simulink model "batteryCellModelling"  (R2024a)
settings: Solver=VariableStepAuto  StartTime=0.0  StopTime=3600  RelTol=1e-3
libraries: fl_lib x7, nesl_utility x4, batteryecm_lib x1
settings Model: Creator=KimoStore  LastModifiedBy=KimoStore
settings ModelReferenceCC: EnableRefExpFcnMdlSchedulingChecks=on
settings RTWCC: GPUComputeCapability=3.5

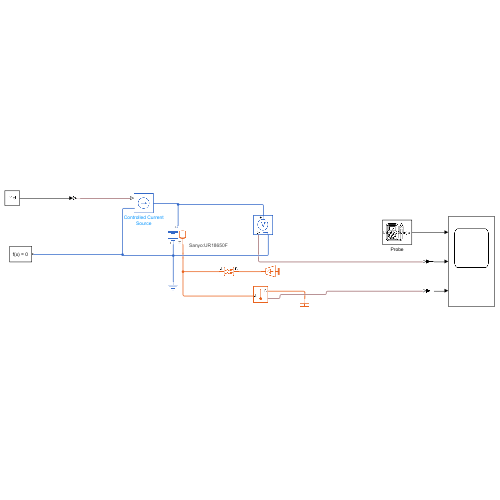
[thumbnail: Simulink's stored preview of the top-level diagram]
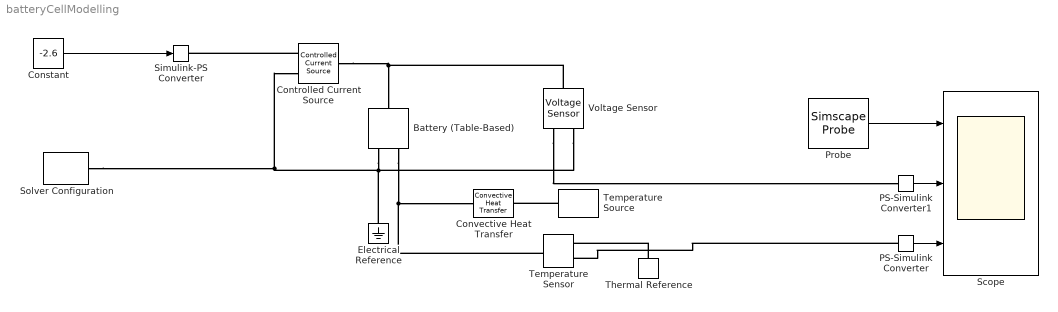
== system batteryCellModelling ==
  Battery (Table-Based) : batteryecm_lib/Battery (Table-Based)  Tag={'toolbox/physmod/battery/shared_library/m/batteryecm_lib_parts';'Battery__Table_Based_/Sanyo/UR18650F.xml'}  SOC_vec=[0 0.01 0.02 0.03 0.04 0.05 0.06 0.07 0.08 0.09 0.1 0.11 0.12 0.13 0.14 0.15 0.16 0.17 0.18 0.19 0.2 0.21 0.22 0.23 0.24 0.25 0.26 0.27 0.28 0.29 0.3 0.31 0.32 0.33 0.34 0.35 0.36 0.37 0.38 0.39 0.4 0.41 0.42 0.43 0.44 0.45 0.46 0.47 0.48 0.49 0.5 0.51 0.52 0.53 0.54 0.55 0.56 0.57 0.58 0.59 0.6 0.61 0.62 0.63 0.64 0.65 0.66 0.67 0.68 0.69 0.7 0.71 0.72 0.73 0.74 0.75 0.76 0.77 0.78 0.79 0.8 0.81 0.82 0.83 0.84 0.85 0.86 0.87 0.88 0.89 0.9 0.91 0.92 0.93 0.94 0.95 0.96 0.97 0.98 0.99 1]  T_dependence=simscape.enum.tablebattery.temperature_dependence.yes  prm_dir=simscape.enum.tablebattery.prm_dir.noCurrentDirectionality  T_vec=[-20 -10 0 20 40] degC  V0_mat=[3.0106 3.0106 3.0106 3.0106 3.0106;3.47625 3.47625 3.47625 3.47625 3.47625;3.60079 3.60079 3.60079 3.60079 3.60079;3.6231 3.6231 3.6231 3.6231 3.6231;3.64643 3.64643 3.64643 3.64643 3.64643;3.64894 3.64894 3.64894 3.64894 3.64894;3.65685 3.65685 3.65685 3.65685 3.65685;3.66356 3.66356 3.66356 3.66356 3.66356;3.66315 3.66315 3.66315 3.66315 3.66315;3.6671 3.6671 3.6671 3.6671 3.6671;3.67003 3.67003 3.67003 3.67003 3.67003;3.67239 3.67239 3.67239 3.67239 3.67239;3.67782 3.67782 3.67782 3.67782 3.67782;3.68366 3.68366 3.68366 3.68366 3.68366;3.68873 3.68873 3.68873 3.68873 3.68873;3.6931 3.6931 3.6931 3.6931 3.6931;3.69764 3.69764 3.69764 3.69764 3.69764;3.70218 3.70218 3.70218 3.70218 3.70218;3.70672 3.70672 3.70672 3.70672 3.70672;3.7109 3.7109 3.7109 3.7109 3.7109;3.71581 3.71581 3.71581 3.71581 3.71581;3.71846 3.71846 3.71846 3.71846 3.71846;3.7202 3.7202 3.7202 3.7202 3.7202;3.72195 3.72195 3.72195 3.72195 3.72195;3.7237 3.7237 3.7237 3.7237 3.7237;3.72544 3.72544 3.72544 3.72544 3.72544;3.72714 3.72714 3.72714 3.72714 3.72714;3.72856 3.72856 3.72856 3.72856 3.72856;3.72994 3.72994 3.72994 3.72994 3.72994;3.73135 3.73135 3.73135 3.73135 3.73135;3.7329 3.7329 3.7329 3.7329 3.7329;3.73481 3.73481 3.73481 3.73481 3.73481;3.73671 3.73671 3.73671 3.73671 3.73671;3.73861 3.73861 3.73861 3.73861 3.73861;3.74052 3.74052 3.74052 3.74052 3.74052;3.74259 3.74259 3.74259 3.74259 3.74259;3.74529 3.74529 3.74529 3.74529 3.74529;3.74799 3.74799 3.74799 3.74799 3.74799;3.75066 3.75066 3.75066 3.75066 3.75066;3.75332 3.75332 3.75332 3.75332 3.75332;3.75598 3.75598 3.75598 3.75598 3.75598;3.75851 3.75851 3.75851 3.75851 3.75851;3.76097 3.76097 3.76097 3.76097 3.76097;3.76344 3.76344 3.76344 3.76344 3.76344;3.76591 3.76591 3.76591 3.76591 3.76591;3.76898 3.76898 3.76898 3.76898 3.76898;3.77223 3.77223 3.77223 3.77223 3.77223;3.77526 3.77526 3.77526 3.77526 3.77526;3.7786 3.7786 3.7786 3.7786 3.7786;3.78229 3.78229 3.78229 3.78229 3.78229;3.78598 3.78598 3.78598 3.78598 3.78598;3.78967 3.78967 3.78967 3.78967 3.78967;3.79335 3.79335 3.79335 3.79335 3.79335;3.79704 3.79704 3.79704 3.79704 3.79704;3.80111 3.80111 3.80111 3.80111 3.80111;3.80653 3.80653 3.80653 3.80653 3.80653;3.81239 3.81239 3.81239 3.81239 3.81239;3.81825 3.81825 3.81825 3.81825 3.81825;3.8241 3.8241 3.8241 3.8241 3.8241;3.82996 3.82996 3.82996 3.82996 3.82996;3.83582 3.83582 3.83582 3.83582 3.83582;3.84168 3.84168 3.84168 3.84168 3.84168;3.84738 3.84738 3.84738 3.84738 3.84738;3.85296 3.85296 3.85296 3.85296 3.85296;3.85814 3.85814 3.85814 3.85814 3.85814;3.86321 3.86321 3.86321 3.86321 3.86321;3.86829 3.86829 3.86829 3.86829 3.86829;3.87336 3.87336 3.87336 3.87336 3.87336;3.87896 3.87896 3.87896 3.87896 3.87896;3.8849 3.8849 3.8849 3.8849 3.8849;3.89135 3.89135 3.89135 3.89135 3.89135;3.8978 3.8978 3.8978 3.8978 3.8978;3.90491 3.90491 3.90491 3.90491 3.90491;3.91294 3.91294 3.91294 3.91294 3.91294;3.92098 3.92098 3.92098 3.92098 3.92098;3.92901 3.92901 3.92901 3.92901 3.92901;3.93705 3.93705 3.93705 3.93705 3.93705;3.94509 3.94509 3.94509 3.94509 3.94509;3.95312 3.95312 3.95312 3.95312 3.95312;3.9617 3.9617 3.9617 3.9617 3.9617;3.97082 3.97082 3.97082 3.97082 3.97082;3.97992 3.97992 3.97992 3.97992 3.97992;3.98896 3.98896 3.98896 3.98896 3.98896;3.99801 3.99801 3.99801 3.99801 3.99801;4.00706 4.00706 4.00706 4.00706 4.00706;4.01633 4.01633 4.01633 4.01633 4.01633;4.02607 4.02607 4.02607 4.02607 4.02607;4.03582 4.03582 4.03582 4.03582 4.03582;4.04554 4.04554 4.04554 4.04554 4.04554;4.05463 4.05463 4.05463 4.05463 4.05463;4.06371 4.06371 4.06371 4.06371 4.06371;4.07279 4.07279 4.07279 4.07279 4.07279;4.08257 4.08257 4.08257 4.08257 4.08257;4.09311 4.09311 4.09311 4.09311 4.09311;4.10365 4.10365 4.10365 4.10365 4.10365;4.11077 4.11077 4.11077 4.11077 4.11077;4.1214 4.1214 4.1214 4.1214 4.1214;4.13525 4.13525 4.13525 4.13525 4.13525;4.14523 4.14523 4.14523 4.14523 4.14523;4.15493 4.15493 4.15493 4.15493 4.15493;4.155 4.155 4.155 4.155 4.155] V  V0_vec=[3.0106 3.47625 3.60079 3.6231 3.64643 3.64894 3.65685 3.66356 3.66315 3.6671 3.67003 3.67239 3.67782 3.68366 3.68873 3.6931 3.69764 3.70218 3.70672 3.7109 3.71581 3.71846 3.7202 3.72195 3.7237 3.72544 3.72714 3.72856 3.72994 3.73135 3.7329 3.73481 3.73671 3.73861 3.74052 3.74259 3.74529 3.74799 3.75066 3.75332 3.75598 3.75851 3.76097 3.76344 3.76591 3.76898 3.77223 3.77526 3.7786 3.78229 3.78598 3.78967 3.79335 3.79704 3.80111 3.80653 3.81239 3.81825 3.8241 3.82996 3.83582 3.84168 3.84738 3.85296 3.85814 3.86321 3.86829 3.87336 3.87896 3.8849 3.89135 3.8978 3.90491 3.91294 3.92098 3.92901 3.93705 3.94509 3.95312 3.9617 3.97082 3.97992 3.98896 3.99801 4.00706 4.01633 4.02607 4.03582 4.04554 4.05463 4.06371 4.07279 4.08257 4.09311 4.10365 4.11077 4.1214 4.13525 4.14523 4.15493 4.155] V  V_range=[2.25 Inf] V  R0_mat=[0.91079 0.64471 0.66005 0.32334 0.22255;0.91079 0.87564 0.84506 0.31805 0.20422;0.91079 0.8329 0.76988 0.27322 0.1707;0.91079 0.79017 0.69471 0.21555 0.13653;0.91079 0.74743 0.61953 0.18044 0.13199;0.91079 0.70469 0.54435 0.15555 0.11839;0.89131 0.66195 0.46917 0.14033 0.11278;0.87183 0.61922 0.40227 0.13004 0.10754;0.85235 0.57648 0.34276 0.1193 0.09921;0.83287 0.53374 0.30357 0.11358 0.0951;0.81339 0.491 0.27082 0.10902 0.09309;0.79391 0.44972 0.25102 0.10452 0.09083;0.77443 0.42218 0.23448 0.10273 0.08991;0.75495 0.40017 0.22136 0.10131 0.08916;0.73547 0.38109 0.21479 0.09982 0.08941;0.71598 0.36438 0.20791 0.09868 0.08984;0.6965 0.34954 0.20223 0.0977 0.09034;0.67702 0.3347 0.1974 0.09672 0.09084;0.65754 0.32449 0.19266 0.09574 0.09135;0.63806 0.31584 0.19038 0.09479 0.09169;0.61858 0.30751 0.18841 0.09475 0.09236;0.5991 0.2982 0.18547 0.09414 0.09204;0.57962 0.28901 0.18213 0.09327 0.0913;0.56014 0.28113 0.17879 0.0924 0.09052;0.54066 0.27326 0.17545 0.09153 0.08974;0.52118 0.26539 0.17294 0.09066 0.08896;0.50169 0.2601 0.17078 0.08979 0.08816;0.48207 0.25588 0.16849 0.08895 0.08724;0.46245 0.25165 0.1662 0.08807 0.0863;0.44825 0.24744 0.16391 0.0872 0.08538;0.43526 0.24328 0.16168 0.08637 0.08451;0.42243 0.23928 0.1596 0.08563 0.0838;0.4096 0.23563 0.15753 0.0849 0.08307;0.39731 0.2331 0.15546 0.08416 0.08226;0.38796 0.23057 0.15417 0.08343 0.08145;0.37869 0.22811 0.15325 0.08282 0.08071;0.36969 0.22592 0.1526 0.08278 0.08024;0.36068 0.22374 0.15195 0.08273 0.07978;0.35167 0.22154 0.15129 0.08269 0.0793;0.34357 0.21934 0.15063 0.08265 0.07881;0.3386 0.21714 0.14997 0.08261 0.07833;0.33357 0.21488 0.14924 0.08254 0.07779;0.32851 0.21333 0.1485 0.08245 0.07722;0.32346 0.21183 0.14775 0.08237 0.07667;0.3184 0.21032 0.147 0.08229 0.07613;0.31361 0.20908 0.1465 0.08237 0.07586;0.30889 0.20791 0.14606 0.08238 0.07566;0.3052 0.20665 0.14553 0.08215 0.07538;0.30233 0.20553 0.14512 0.08199 0.07522;0.29961 0.20455 0.14487 0.0819 0.07521;0.2969 0.20352 0.14462 0.08181 0.07521;0.29418 0.20224 0.14437 0.08172 0.0752;0.29146 0.20096 0.14411 0.08164 0.0752;0.28874 0.19968 0.14386 0.08155 0.07519;0.28619 0.19857 0.14378 0.08154 0.07489;0.28423 0.19804 0.14428 0.08183 0.07492;0.28246 0.19771 0.14418 0.08218 0.07514;0.2815 0.19737 0.14398 0.08253 0.07536;0.28054 0.19704 0.14379 0.08288 0.07558;0.27959 0.1967 0.14359 0.08324 0.07581;0.27863 0.19637 0.1434 0.08359 0.07603;0.27767 0.1963 0.1432 0.08394 0.07625;0.27665 0.19618 0.14294 0.08429 0.0762;0.27557 0.19601 0.14262 0.08465 0.07583;0.27432 0.19566 0.14213 0.08464 0.07527;0.27302 0.19527 0.1416 0.08454 0.07468;0.27214 0.19488 0.14106 0.08444 0.07408;0.27154 0.19448 0.14052 0.08435 0.07348;0.27116 0.19432 0.14024 0.08439 0.07311;0.27093 0.19408 0.14017 0.08453 0.07289;0.27092 0.19404 0.14033 0.08463 0.07289;0.27091 0.194 0.14049 0.08473 0.07281;0.27118 0.19425 0.14093 0.08499 0.07252;0.27187 0.1949 0.14177 0.08555 0.07263;0.27344 0.19555 0.14262 0.08612 0.07274;0.27564 0.1962 0.14346 0.08668 0.07284;0.27783 0.19685 0.14431 0.08725 0.07295;0.28002 0.19746 0.14514 0.08781 0.07306;0.28222 0.19799 0.14583 0.08838 0.07317;0.28465 0.19876 0.14675 0.08907 0.07352;0.28731 0.19977 0.14791 0.08989 0.07409;0.29048 0.20076 0.14906 0.0907 0.07466;0.29372 0.20197 0.15018 0.09146 0.07473;0.29697 0.205 0.15131 0.09221 0.07474;0.30021 0.20804 0.15243 0.09297 0.07474;0.30355 0.21117 0.15365 0.09374 0.07485;0.30987 0.21451 0.15499 0.09451 0.07516;0.31753 0.21784 0.15619 0.09529 0.07547;0.32517 0.22155 0.15739 0.09605 0.07577;0.33254 0.22644 0.15831 0.09625 0.07551;0.34616 0.23132 0.15922 0.09645 0.07483;0.36274 0.23621 0.16013 0.09665 0.07414;0.37963 0.2429 0.16135 0.097 0.07376;0.39684 0.25082 0.16268 0.09751 0.07371;0.41405 0.25875 0.1638 0.09803 0.07365;0.43741 0.26477 0.16344 0.0954 0.07088;0.46638 0.26422 0.16461 0.09327 0.06933;0.48546 0.26468 0.16425 0.09123 0.06918;0.48727 0.25441 0.15953 0.08483 0.06734;0.46461 0.24401 0.14595 0.07819 0.06447;0.3977 0.19886 0.12275 0.06301 0.03811] Ohm  R0_vec=[0.32334 0.31805 0.27322 0.21555 0.18044 0.15555 0.14033 0.13004 0.1193 0.11358 0.10902 0.10452 0.10273 0.10131 0.09982 0.09868 0.0977 0.09672 0.09574 0.09479 0.09475 0.09414 0.09327 0.0924 0.09153 0.09066 0.08979 0.08895 0.08807 0.0872 0.08637 0.08563 0.0849 0.08416 0.08343 0.08282 0.08278 0.08273 0.08269 0.08265 0.08261 0.08254 0.08245 0.08237 0.08229 0.08237 0.08238 0.08215 0.08199 0.0819 0.08181 0.08172 0.08164 0.08155 0.08154 0.08183 0.08218 0.08253 0.08288 0.08324 0.08359 0.08394 0.08429 0.08465 0.08464 0.08454 0.08444 0.08435 0.08439 0.08453 0.08463 0.08473 0.08499 0.08555 0.08612 0.08668 0.08725 0.08781 0.08838 0.08907 0.08989 0.0907 0.09146 0.09221 0.09297 0.09374 0.09451 0.09529 0.09605 0.09625 0.09645 0.09665 0.097 0.09751 0.09803 0.0954 0.09327 0.09123 0.08483 0.07819 0.06301] Ohm  R0_dis_mat=[.0117, .0085, .009; .011, .0085, .009; .0114, .0087, .0092; .0107, .0082, .0088; .0107, .0083, .0091; .0113, .0085, .0089; .0116, .0085, .0089] % Parameter not set Ohm  R0_dis_vec=[.0085, .0085, .0087, .0082, .0083, .0085, .0085] % Parameter not set Ohm  R0_ch_mat=[.0117, .0085, .009; .011, .0085, .009; .0114, .0087, .0092; .0107, .0082, .0088; .0107, .0083, .0091; .0113, .0085, .0089; .0116, .0085, .0089] % Parameter not set Ohm  R0_ch_vec=[.0085, .0085, .0087, .0082, .0083, .0085, .0085] % Parameter not set Ohm  AH=2.396 hr*A  prm_leak=simscape.enum.tablebattery.prm_leak.disabled  Rleak_vec=[8000, 7000, 6000] % Parameter not set Ohm  Rleak=7e3 % Parameter not set Ohm  extrapolation_option=simscape.enum.extrapolation.nearest  SOC_port=simscape.enum.tablebattery.enable.no  prm_dyn=simscape.enum.tablebattery.prm_dyn.off  R1_mat=[.0109, .0029, .0013; .0069, .0024, .0012; .0047, .0026, .0013; .0034, .0016, .001; .0033, .0023, .0014; .0033, .0018, .0011; .0028, .0017, .0011] % Parameter not set Ohm  R1_vec=[.0029, .0024, .0026, .0016, .0023, .0018, .0017] % Parameter not set Ohm  tau1_mat=[20, 36, 39; 31, 45, 39; 109, 105, 61; 36, 29, 26; 59, 77, 67; 40, 33, 29; 25, 39, 33] % Parameter not set s  tau1_vec=[36, 45, 105, 29, 77, 33, 39] % Parameter not set s  R2_mat=[.0109, .0029, .0013; .0069, .0024, .0012; .0047, .0026, .0013; .0034, .0016, .001; .0033, .0023, .0014; .0033, .0018, .0011; .0028, .0017, .0011] % Parameter not set Ohm  R2_vec=[.0029, .0024, .0026, .0016, .0023, .0018, .0017] % Parameter not set Ohm  tau2_mat=[20, 36, 39; 31, 45, 39; 109, 105, 61; 36, 29, 26; 59, 77, 67; 40, 33, 29; 25, 39, 33] % Parameter not set s  tau2_vec=[36, 45, 105, 29, 77, 33, 39] % Parameter not set s  R3_mat=[.0109, .0029, .0013; .0069, .0024, .0012; .0047, .0026, .0013; .0034, .0016, .001; .0033, .0023, .0014; .0033, .0018, .0011; .0028, .0017, .0011] % Parameter not set Ohm  R3_vec=[.0029, .0024, .0026, .0016, .0023, .0018, .0017] % Parameter not set Ohm  tau3_mat=[20, 36, 39; 31, 45, 39; 109, 105, 61; 36, 29, 26; 59, 77, 67; 40, 33, 29; 25, 39, 33] % Parameter not set s  tau3_vec=[36, 45, 105, 29, 77, 33, 39] % Parameter not set s  R4_mat=[.0109, .0029, .0013; .0069, .0024, .0012; .0047, .0026, .0013; .0034, .0016, .001; .0033, .0023, .0014; .0033, .0018, .0011; .0028, .0017, .0011] % Parameter not set Ohm  R4_vec=[.0029, .0024, .0026, .0016, .0023, .0018, .0017] % Parameter not set Ohm  tau4_mat=[20, 36, 39; 31, 45, 39; 109, 105, 61; 36, 29, 26; 59, 77, 67; 40, 33, 29; 25, 39, 33] % Parameter not set s  tau4_vec=[36, 45, 105, 29, 77, 33, 39] % Parameter not set s  R5_mat=[.0109, .0029, .0013; .0069, .0024, .0012; .0047, .0026, .0013; .0034, .0016, .001; .0033, .0023, .0014; .0033, .0018, .0011; .0028, .0017, .0011] % Parameter not set Ohm  R5_vec=[.0029, .0024, .0026, .0016, .0023, .0018, .0017] % Parameter not set Ohm  tau5_mat=[20, 36, 39; 31, 45, 39; 109, 105, 61; 36, 29, 26; 59, 77, 67; 40, 33, 29; 25, 39, 33] % Parameter not set s  tau5_vec=[36, 45, 105, 29, 77, 33, 39] % Parameter not set s  prm_fade=simscape.enum.tablebattery.prm_fade.tableN  N0=100 % Parameter not set  dV0=0 % Parameter not set  dR0=0 % Parameter not set  dAH=0 % Parameter not set  dRleak=0 % Parameter not set  dR1=0 % Parameter not set  dR2=0 % Parameter not set  dR3=0 % Parameter not set  dR4=0 % Parameter not set  dR5=0 % Parameter not set  N0vec=[0 6 11 16 21 26 31 36 41 46 51 56 61 66 71 76 81 86 91 96 101 106 111 116 121 126 131 136 141 146 151 156 161 166 171 176 181 186 191 196 201 206 211 216 221 226 231 236 241 246 251 256 261 266 271 276 281 286 291 296 301 306 311 316 321 326 331 336 341 346 351 356 361 366 371 376 381 386 391 396 401 406 411 416 421 426 431 436 441 446 451 456 461 466 471 476 481 486 491 496]  Tfadevec=[298.15, 323.15] % Parameter not set K  dV0vec=[0 -0.0008 -0.0017 -0.1142 -0.2296 -0.348 -0.4665 -0.5391 -0.6153 -0.6915 -0.7677 -0.8357 -0.8941 -0.9526 -1.0196 -1.0824 -1.1303 -1.1783 -1.2262 -1.2925 -1.3557 -1.4144 -1.4731 -1.5319 -1.5906 -1.6493 -1.7081 -1.7651 -1.8196 -1.8742 -1.9287 -1.9828 -2.0331 -2.0834 -2.1337 -2.184 -2.2343 -2.2846 -2.3349 -2.3852 -2.4355 -2.4859 -2.5362 -2.5866 -2.6371 -2.691 -2.7432 -2.7949 -2.8466 -2.8984 -2.9501 -3.0019 -3.0537 -3.1055 -3.1573 -3.209 -3.2565 -3.301 -3.3452 -3.3875 -3.4299 -3.4722 -3.5146 -3.5569 -3.5984 -3.6397 -3.681 -3.7224 -3.7675 -3.8137 -3.8599 -3.9061 -3.9523 -3.9985 -4.0447 -4.0909 -4.137 -4.1832 -4.2288 -4.2723 -4.3158 -4.3593 -4.4028 -4.4463 -4.4899 -4.5334 -4.577 -4.6205 -4.6634 -4.7044 -4.7484 -4.7927 -4.8369 -4.8797 -4.9212 -4.9626 -5.004 -5.0455 -5.0869 -5.1283]  dR0vec=[0 0 0 0 0 0 0 0 0 0 0 0 0 0 0 0 0 0 0 0 0 0 0 0 0 0 0 0 0 0 0 0 0 0 0 0 0 0 0 0 0 0 0 0 0 0 0 0 0 0 0 0 0 0 0 0 0 0 0 0 0 0 0 0 0 0 0 0 0 0 0 0 0 0 0 0 0 0 0 0 0 0 0 0 0 0 0 0 0 0 0 0 0 0 0 0 0 0 0 0] % Parameter assumed  dAHvec=[0 -0.494 -0.988 -1.482 -1.975 -2.469 -2.962 -3.191 -3.42 -3.648 -3.877 -4.105 -4.334 -4.562 -4.824 -5.104 -5.384 -5.663 -5.943 -6.223 -6.472 -6.703 -6.935 -7.167 -7.398 -7.63 -7.861 -8.093 -8.325 -8.556 -8.788 -9.019 -9.249 -9.479 -9.709 -9.94 -10.17 -10.4 -10.63 -10.86 -11.091 -11.321 -11.551 -11.781 -12.011 -12.242 -12.465 -12.686 -12.906 -13.127 -13.348 -13.569 -13.79 -14.01 -14.231 -14.452 -14.654 -14.844 -15.034 -15.224 -15.414 -15.604 -15.793 -15.983 -16.173 -16.363 -16.553 -16.743 -16.95 -17.162 -17.374 -17.586 -17.799 -18.011 -18.223 -18.435 -18.647 -18.859 -19.068 -19.267 -19.465 -19.664 -19.863 -20.061 -20.26 -20.458 -20.657 -20.855 -21.054 -21.252 -21.466 -21.68 -21.894 -22.108 -22.323 -22.537 -22.751 -22.965 -23.18 -23.394]  dRleakvec=[0, 0, 0, 0] % Parameter not set  dR1vec=[0, 0, 0, 0] % Parameter not set  dR2vec=[0, 0, 0, 0] % Parameter not set  dR3vec=[0, 0, 0, 0] % Parameter not set  dR4vec=[0, 0, 0, 0] % Parameter not set  dR5vec=[0, 0, 0, 0] % Parameter not set  dV0mat=[0, 0; 0, 0; 0, 0; 0, 0] % Parameter not set  dR0mat=[0, 0; 0, 0; 0, 0; 0, 0] % Parameter not set  dAHmat=[0, 0; 0, 0; 0, 0; 0, 0] % Parameter not set  dRleakmat=[0, 0; 0, 0; 0, 0; 0, 0] % Parameter not set  dR1mat=[0, 0; 0, 0; 0, 0; 0, 0] % Parameter not set  dR2mat=[0, 0; 0, 0; 0, 0; 0, 0] % Parameter not set  dR3mat=[0, 0; 0, 0; 0, 0; 0, 0] % Parameter not set  dR4mat=[0, 0; 0, 0; 0, 0; 0, 0] % Parameter not set  dR5mat=[0, 0; 0, 0; 0, 0; 0, 0] % Parameter not set  prm_age_modeling=simscape.enum.tablebattery.prm_age_modeling.equation  storage_dt_age_vec=[0] % Parameter not set d  storage_T_age_vec=[273] % Parameter not set K  prm_age_OCV=simscape.enum.tablebattery.prm_age_OCV.OCV  OCV_age=0.9 % Parameter not set  SOC_age=0.6 % Parameter not set  prm_age_resistance=simscape.enum.tablebattery.prm_age.disabled  OCV_scaling_age_resistance=2.2134e6 % Parameter not set  OCV_offset_age_resistance=1.632e6 % Parameter not set  temp_exp_age_resistance=0.515833569 % Parameter not set V  t_exp_age_resistance=0.75 % Parameter not set  T_age_vec_resistance=[273.15, 298.15, 323.15] % Parameter not set K  dt_age_vec_resistance=[0, 90, 180, 270] % Parameter not set d  dR0_age_vec=[0, 0, 0] % Parameter not set  t_meas_dR0_age=100 % Parameter not set d  dR0_age_mat=[0, 0, 0; 0, 0, 0; 0, 0, 0; 0, 0, 0] % Parameter not set  prm_age_capacity=simscape.enum.tablebattery.prm_age.disabled  OCV_scaling_age_capacity=1.5097e07 % Parameter not set  OCV_offset_age_capacity=8.3625e06 % Parameter not set  temp_exp_age_capacity=0.6011 % Parameter not set V  t_exp_age_capacity=0.75 % Parameter not set  T_age_vec_capacity=[273.15, 298.15, 323.15] % Parameter not set K  dt_age_vec_capacity=[0, 90, 180, 270] % Parameter not set d  dAH_age_vec=[0, 0, 0] % Parameter not set  t_meas_dAH_age=100 % Parameter not set d  dAH_age_mat=[0, 0, 0; 0, 0, 0; 0, 0, 0; 0, 0, 0] % Parameter not set  thermal_port=simscape.enum.thermaleffects.model  temperature=298.15 % Parameter not set K  thermal_mass=40.05 % Parameter assumed J/K  i_specify=off  i_priority=None  i=0 A  i_nominal_specify=off  i_nominal_value=1  i_nominal_unit=A  v_specify=off  v_priority=None  v=0 V  v_nominal_specify=off  v_nominal_value=1  v_nominal_unit=V  stateOfCharge_specify=on  stateOfCharge_priority=High  stateOfCharge=1  stateOfCharge_nominal_specify=on  stateOfCharge_nominal_value=1  stateOfCharge_nominal_unit=1  num_cycles_specify=off  num_cycles_priority=High  num_cycles=0  num_cycles_nominal_specify=off  num_cycles_nominal_value=1  num_cycles_nominal_unit=1  cell_temperature_specify=off  cell_temperature_priority=High  cell_temperature=298.15 K  cell_temperature_nominal_specify=off  cell_temperature_nominal_value=1  cell_temperature_nominal_unit=K
      settings: AttributesFormatString=Sanyo:UR18650F  InternalSimscapePortConfiguration="{\"Bottom\":[],\"Left\":[{\"id\":\"p\",\"label\":\"+\",\"type\":\"foundation.electrical.electrical\"}],\"Right\":[{\"id\":\"n\",\"label\":\"-\",\"type\":\"foundation.electrical.electrical\"},{\"id\":\"H\",\"label\":\"H\",\"type\":\"foundation.thermal.thermal\"}],\"Top\":[]}"
  Constant : Constant  Value=-2.6
  Controlled Current Source : fl_lib/Electrical/Electrical Sources/Controlled Current Source
  Convective Heat Transfer : fl_lib/Thermal/Thermal Elements/Convective Heat Transfer  thermal_type=foundation.enum.constant_variable.constant  area=1e-4 m^2  heat_tr_coeff=20 W/(K*m^2)  min_heat_tr_coeff=1e-3 W/(K*m^2)  T_specify=off  T_priority=None  T=0 K  T_nominal_specify=off  T_nominal_value=1  T_nominal_unit=K  Q_specify=off  Q_priority=None  Q=0 W  Q_nominal_specify=off  Q_nominal_value=1  Q_nominal_unit=W
  Electrical Reference : fl_lib/Electrical/Electrical Elements/Electrical Reference
  PS-Simulink Converter : nesl_utility/PS-Simulink Converter  PhysicalDomain=network_engine_domain  SubClassName=ps_output  LeftPortType=input  RightPortType=output  PseudoPeriodic=off  Frequencies=[]  VectorFormat=inherit  Unit=inherit  AffineConversion=off
  PS-Simulink Converter1 : nesl_utility/PS-Simulink Converter  PhysicalDomain=network_engine_domain  SubClassName=ps_output  LeftPortType=input  RightPortType=output  PseudoPeriodic=off  Frequencies=[]  VectorFormat=inherit  Unit=inherit  AffineConversion=off
  Probe : SimscapeProbe  BoundBlock=9  Variables={stateOfCharge}
  Scope : Scope  NumInputPorts=3
  Simulink-PS Converter : nesl_utility/Simulink-PS Converter  PhysicalDomain=network_engine_domain  SubClassName=ps_input  LeftPortType=input  RightPortType=output  PseudoPeriodic=off  Frequencies=[]  NoiseDistribution=none  NoiseParameters=[]  Unit=1  AffineConversion=off  FilteringAndDerivatives=provide  SimscapeFilterOrder=1  InputFilterTimeConstant=0.001  UdotUserProvided=0
  Solver Configuration : nesl_utility/Solver Configuration  PhysicalDomain=network_engine_domain  SubClassName=solver  LeftPortType=input  RightPortType=generic  Tones=[]  Harmonics=[]  SimulateNoise=off  Profile=off  UseLocalSampling=off  EnableSwitchedLinearOptims=on  FrequencyDomain=off  UseCCode=off  RelTol=0.001  AbsTol=0.001  MinStep=1e-09  ToWorkspace=off  RevertToSquareIcSolve=off  NumHomotopyIterations=100  PhasorMode=off  PhasorModeNumHarmonics=1  ConsistencySolver=NEWTON_FTOL  IndexReductionMethod=DerivativeReplacement  DoDC=off  ResidualTolerance=1e-09  ConsistencyTolSource=GLOBAL  ConsistencyAbsTol=0.001  ConsistencyRelTol=0.001  ConsistencyTolFactor=0.001  UseLocalSolver=off  LocalSolverChoice=NE_BACKWARD_EULER_ADVANCER  ResolveIndetEquations=on  FunctionEvalNumThread=1  LocalSolverSampleTime=0.001  DoFixedCost=off  MaxNonlinIter=3  MaxModeIter=2  ComputeImpulses=off  ImpulseIterations=2  LinearAlgebra=auto  LinearAlgebraNumThread=0  EquationFormulation=NE_TIME_EF  DelaysMemoryBudget=1024  AutomaticFiltering=on  FilteringTimeConstant=0.001  PartitionStorageMethod=AS_NEEDED  PartitionMemoryBudget=1024  PartitionMethod=ROBUST  MultibodyUseLocalSolver=off  MultibodyLocalSolverChoice=ODE1  MultibodyLocalSolverSampleTime=0.001
  Temperature Sensor : fl_lib/Thermal/Thermal Sensors/Temperature Sensor  temperature_measure=foundation.enum.MeasurementReference.difference
  Temperature Source : fl_lib/Thermal/Thermal Sources/Temperature Source  temperature=293.15 K
  Thermal Reference : fl_lib/Thermal/Thermal Elements/Thermal Reference
  Voltage Sensor : fl_lib/Electrical/Electrical Sensors/Voltage Sensor
  wires:
  Constant/1 -> Simulink-PS Converter/1
  PS-Simulink Converter/1 -> Scope/3
  PS-Simulink Converter1/1 -> Scope/2
  Probe/1 -> Scope/1
  connections:
  Controlled Current Source/RConn1 -- Simulink-PS Converter/RConn1
  Controlled Current Source/LConn1 -- Voltage Sensor/LConn1 -- Battery (Table-Based)/LConn1
  Battery (Table-Based)/RConn1 -- Electrical Reference/LConn1 -- Solver Configuration/RConn1 -- Controlled Current Source/RConn2 -- Voltage Sensor/RConn2
  Battery (Table-Based)/RConn2 -- Temperature Sensor/LConn1 -- Convective Heat Transfer/LConn1
  Temperature Source/LConn1 -- Convective Heat Transfer/RConn1
  Thermal Reference/LConn1 -- Temperature Sensor/RConn1
  PS-Simulink Converter/LConn1 -- Temperature Sensor/RConn2
  Voltage Sensor/RConn1 -- PS-Simulink Converter1/LConn1
